simulink model "vestibular_3GDL"  (Simulink 7.7)
settings: Solver=ode45  StartTime=0.0  StopTime=30  RelTol=1e-3
values from neighbouring files (symbols this model uses):
  J = 0.02    [DCmotor.m]    (also in constantes_robot.m)
  Kb = 0.1    [DCmotor.m]    (also in constantes_robot.m)
  Kf = 0.2    [DCmotor.m]    (also in constantes_robot.m)
  Kff = 1/dcgain(dcm(1))    [DCmotor.m]    (also in constantes_robot.m)
  ki = str2double(get(hObject,'String'))    [interfaz_grafica.m]    (also in robot_simulacion.m = 8)
  ki1 = str2double(get(hObject,'String'))    [interfaz_grafica.m]    (also in robot_simulacion.m = 8)
  Km = 0.1    [DCmotor.m]    (also in constantes_robot.m)
  kp = str2double(get(hObject,'String'))    [interfaz_grafica.m]    (also in robot_simulacion.m = 2)
  L = 0.5    [DCmotor.m]    (also in constantes_robot.m)
  m = 1070    [constantesvestibular.m]    (also in modelo_vestibular.m)
  R = 2.0    (= 2)    [DCmotor.m]    (also in constantes_robot.m)
undefined symbols (not defined in the file or in its folder): articulacionX, articulacionY2, base, cabezalter, mastil, plataforma3, RootGround, RootPart, sigbuilder_block, vestibular_3GDL
libraries: mblibv1 x30, simulink_extras x3
settings Model: Creator=Ángel  LastModifiedBy=Ángel
settings SimMechanicsCC: VisOnUpdateDiagram=on  VisDuringSimulation=on

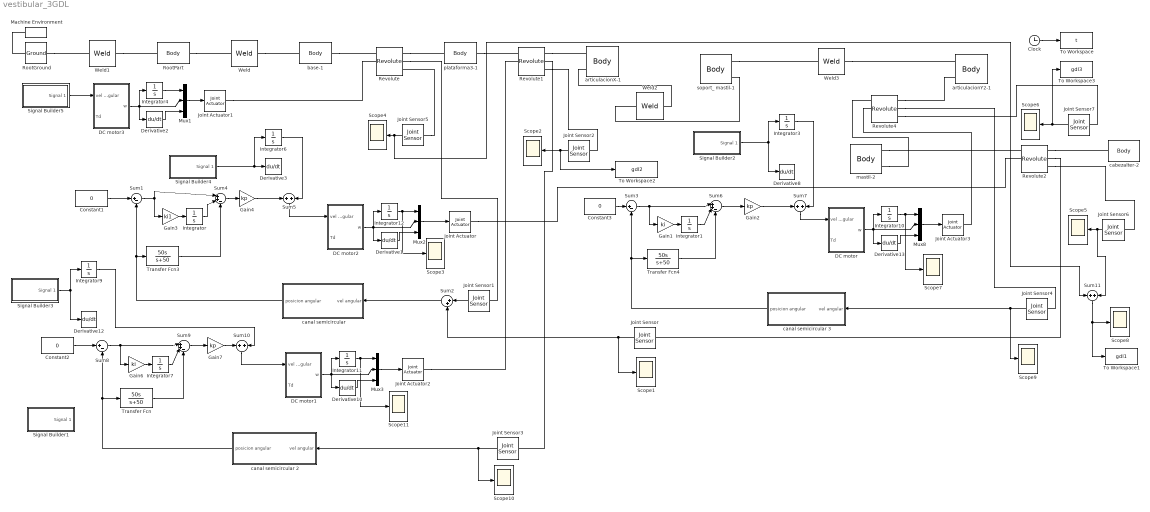
== system vestibular_3GDL ==
  Clock : Clock
      settings: Decimation=10
  Constant1 : Constant  Value=0
  Constant2 : Constant  Value=0
  Constant3 : Constant  Value=0
  DC motor : Subsystem
  DC motor1 : Subsystem
  DC motor2 : Subsystem
  DC motor3 : Subsystem
  Derivative{1..3,8,10,12..13} (7 alike) : Derivative
  Gain1 : Gain  Gain=ki
  Gain2 : Gain  Gain=kp
  Gain3 : Gain  Gain=ki1
  Gain4 : Gain  Gain=kp
  Gain6 : Gain  Gain=ki
  Gain7 : Gain  Gain=kp
  Integrator{,1,3..4,6..7,9..12} (10 alike) : Integrator
  Joint Actuator{,1..3} (4 alike) : mblibv1/Sensors &  Actuators/Joint Actuator  SystemSampleTime=-1  UpdateFromCAD=off  PhysicalDomain=Mechanical  PortType=blob  ActuationStyle=Motion  AngleUnits=rad  ArcVelocityUnits=rad/s  ArcAccelerationUnits=rad/s^2  CoordPositionUnits=m  VelocityUnits=m/s  AccelerationUnits=m/s^2  ForceUnits=N  TorqueUnits=N*m  ActiveIO=on  Width=3  DialogClass=MechanicalActuatorBlock  Primitive=R1  ReferenceFrame=Absolute (World)
  Joint Sensor : mblibv1/Sensors &  Actuators/Joint Sensor  SystemSampleTime=-1  UpdateFromCAD=off  PhysicalDomain=Mechanical  PortType=blob  Muxed=on  Pose=off  Angle=off  AngleUnits=rad  ArcVelocity=on  ArcVelocityUnits=rad/s  ArcAcceleration=off  ArcAccelerationUnits=deg/s^2  CoordPosition=on  CoordPositionUnits=m  Velocity=off  VelocityUnits=m/s  Acceleration=off  AccelerationUnits=m/s^2  Quaternion=on  QuaternionDT=off  QuaternionDDT=off  QuaternionUnits=off  OutputVector=[1]  ActiveIO=on  Width=1  DialogClass=MechanicalSensorBlock  Primitive=R1  Force=off  ForceUnits=N  Torque=off  TorqueUnits=N*m  ReferenceFrame=Absolute (World)  ReactionSensedSide=Base  ReactionReferenceFrame=Absolute (World)  ReactionForce=off  ReactionForceUnits=N  ReactionMoment=off  ReactionMomentUnits=N*m
  Joint Sensor1 : mblibv1/Sensors &  Actuators/Joint Sensor  SystemSampleTime=-1  UpdateFromCAD=off  PhysicalDomain=Mechanical  PortType=blob  Muxed=on  Pose=off  Angle=off  AngleUnits=rad  ArcVelocity=on  ArcVelocityUnits=rad/s  ArcAcceleration=off  ArcAccelerationUnits=rad/s^2  CoordPosition=on  CoordPositionUnits=m  Velocity=off  VelocityUnits=m/s  Acceleration=off  AccelerationUnits=m/s^2  Quaternion=on  QuaternionDT=off  QuaternionDDT=off  QuaternionUnits=off  OutputVector=[1]  ActiveIO=on  Width=1  DialogClass=MechanicalSensorBlock  Primitive=R1  Force=off  ForceUnits=N  Torque=off  TorqueUnits=N*m  ReferenceFrame=Absolute (World)  ReactionSensedSide=Base  ReactionReferenceFrame=Absolute (World)  ReactionForce=off  ReactionForceUnits=N  ReactionMoment=off  ReactionMomentUnits=N*m
  Joint Sensor{2,5..7} (4 alike) : mblibv1/Sensors &  Actuators/Joint Sensor  SystemSampleTime=-1  UpdateFromCAD=off  PhysicalDomain=Mechanical  PortType=blob  Muxed=on  Pose=off  Angle=on  AngleUnits=deg  ArcVelocity=off  ArcVelocityUnits=rad/s  ArcAcceleration=off  ArcAccelerationUnits=rad/s^2  CoordPosition=on  CoordPositionUnits=m  Velocity=off  VelocityUnits=m/s  Acceleration=off  AccelerationUnits=m/s^2  Quaternion=on  QuaternionDT=off  QuaternionDDT=off  QuaternionUnits=off  OutputVector=[1]  ActiveIO=on  Width=1  DialogClass=MechanicalSensorBlock  Primitive=R1  Force=off  ForceUnits=N  Torque=off  TorqueUnits=N*m  ReferenceFrame=Absolute (World)  ReactionSensedSide=Base  ReactionReferenceFrame=Absolute (World)  ReactionForce=off  ReactionForceUnits=N  ReactionMoment=off  ReactionMomentUnits=N*m
  Joint Sensor3 : mblibv1/Sensors &  Actuators/Joint Sensor  SystemSampleTime=-1  UpdateFromCAD=off  PhysicalDomain=Mechanical  PortType=blob  Muxed=on  Pose=off  Angle=off  AngleUnits=rad  ArcVelocity=on  ArcVelocityUnits=rad/s  ArcAcceleration=off  ArcAccelerationUnits=rad/s^2  CoordPosition=on  CoordPositionUnits=m  Velocity=off  VelocityUnits=m/s  Acceleration=off  AccelerationUnits=m/s^2  Quaternion=on  QuaternionDT=off  QuaternionDDT=off  QuaternionUnits=off  OutputVector=[1]  ActiveIO=on  Width=1  DialogClass=MechanicalSensorBlock  Primitive=R1  Force=off  ForceUnits=N  Torque=off  TorqueUnits=N*m  ReferenceFrame=Absolute (World)  ReactionSensedSide=Base  ReactionReferenceFrame=Absolute (World)  ReactionForce=off  ReactionForceUnits=N  ReactionMoment=off  ReactionMomentUnits=N*m
  Joint Sensor4 : mblibv1/Sensors &  Actuators/Joint Sensor  SystemSampleTime=-1  UpdateFromCAD=off  PhysicalDomain=Mechanical  PortType=blob  Muxed=on  Pose=off  Angle=off  AngleUnits=rad  ArcVelocity=on  ArcVelocityUnits=rad/s  ArcAcceleration=off  ArcAccelerationUnits=rad/s^2  CoordPosition=on  CoordPositionUnits=m  Velocity=off  VelocityUnits=m/s  Acceleration=off  AccelerationUnits=m/s^2  Quaternion=on  QuaternionDT=off  QuaternionDDT=off  QuaternionUnits=off  OutputVector=[1]  ActiveIO=on  Width=1  DialogClass=MechanicalSensorBlock  Primitive=R1  Force=off  ForceUnits=N  Torque=off  TorqueUnits=N*m  ReferenceFrame=Absolute (World)  ReactionSensedSide=Base  ReactionReferenceFrame=Absolute (World)  ReactionForce=off  ReactionForceUnits=N  ReactionMoment=off  ReactionMomentUnits=N*m
  Machine Environment : mblibv1/Bodies/Machine Environment  SystemSampleTime=-1  PortType=env  PhysicalDomain=Mechanical  DialogTemplateClass=MECH.MachineEnvironment  SyncWhenCopied=off  Gravity=[0 -9.81 0]  GravityUnits=m/s^2  GravityAsSignal=off  Dimensionality=Auto-detect  AnalysisType=Forward dynamics  LinearAssemblyTolerance=1e-3  LinearAssemblyToleranceUnits=m  AngularAssemblyTolerance=1e-3  AngularAssemblyToleranceUnits=rad  ConstraintSolverType=Stabilizing  ConstraintRelTolerance=1e-4  ConstraintAbsTolerance=1e-4  UseRobustSingularityHandling=off  RedundancyAnalysisToleranceType=Automatically select tolerance  RedundancyAnalysisTolerance=1e-14  StatePerturbationType=Fixed  PerturbationSize=1e-5  VisualizeMachine=on  BodyVisualizationType=Use model default body geometries  BodyColorSelMode=Use model default  DefaultBodyColor=[1 0 0]
  Mux{1..3,8} (4 alike) : Mux  Inputs=3
  Revolute : mblibv1/Joints/Revolute  PhysicalDomain=mechanical  SubClassName=Unknown  LeftPortType=blob  RightPortType=blob  LConnTagsString=__newl0|SA1|SA2  RConnTagsString=__newr0|SA1|SA2  UpdateFromCAD=on  PMImportedID=base-1:-:plataforma3-1  NumSAPorts=4  CutJoint=off  MarkAsCut=off  Primitives=prismatic  PrimitiveProps=R1$World$[-0.196775,0.962005,-0.189279]$revolute  DialogClass=JointBlock  R1Axis=[-0.196775,0.962005,-0.189279]
  Revolute1 : mblibv1/Joints/Revolute  PhysicalDomain=mechanical  SubClassName=Unknown  LeftPortType=blob  RightPortType=blob  LConnTagsString=__newl0|SA1|SA2  RConnTagsString=__newr0|SA1|SA2  UpdateFromCAD=on  PMImportedID=articulacionX-1:-:plataforma3-1  NumSAPorts=4  CutJoint=off  MarkAsCut=off  Primitives=prismatic  PrimitiveProps=R1$World$[-0.092947,-0.210487,-0.973168]$revolute  DialogClass=JointBlock  R1Axis=[-0.092947,-0.210487,-0.973168]
  Revolute2 : mblibv1/Joints/Revolute  PhysicalDomain=mechanical  SubClassName=Unknown  LeftPortType=blob  RightPortType=blob  LConnTagsString=__newl0|SA1|SA2  RConnTagsString=__newr0|SA1|SA2  UpdateFromCAD=on  PMImportedID=cabezalter-2:-:mastil-2  NumSAPorts=4  CutJoint=off  MarkAsCut=off  Primitives=prismatic  PrimitiveProps=R1$World$[-0.196775,0.962005,-0.189279]$revolute  DialogClass=JointBlock  R1Axis=[-0.196775,0.962005,-0.189279]
  Revolute4 : mblibv1/Joints/Revolute  PhysicalDomain=mechanical  SubClassName=Unknown  LeftPortType=blob  RightPortType=blob  LConnTagsString=__newl0|SA1|SA2  RConnTagsString=__newr0|SA1|SA2  UpdateFromCAD=on  PMImportedID=articulacionY2-1:-:mastil-2  NumSAPorts=4  CutJoint=off  MarkAsCut=off  Primitives=prismatic  PrimitiveProps=R1$World$[-0.976033,-0.173903,0.130834]$revolute  DialogClass=JointBlock  R1Axis=[-0.976033,-0.173903,0.130834]
  RootGround : mblibv1/Bodies/Ground  SystemSampleTime=-1  UpdateFromCAD=on  PMImportedID=RootGround  LeftPortType=env  RightPortType=workingframe  PhysicalDomain=Mechanical  DialogClass=GroundBlock  CoordPosition=[-0.906757,1.13031,1.7432]  CoordPositionUnits=m  StateVectorMgrId=-1  MachineId=[0 0]  ShowEnvPort=on
  RootPart : mblibv1/Bodies/Body  PhysicalDomain=mechanical  SubClassName=Unknown  LeftPortType=workingframe  RightPortType=workingframe  LConnTagsString=CS3  RConnTagsString=CS2  UpdateFromCAD=on  PMImportedID=vestibular_3GDL/RootPart  DialogClass=MechanicalBodyBlock  Mass=0  MassUnits=kg  InertiaUnits=kg*m^2  Inertia=[0,0,0;0,0,0;0,0,0]  Shape=Cylinder  ShapeDims=[1 1]  ShapeUnits=m  ShapeUse=false  Density=1  DensityUnits=kg/m^3  DensityUse=false  GraphicsMode=MACHINE_DEFAULT  BodyColorSelMode=MACHINE_DEFAULT  BodyColor=[1;0;0]  AttachedToCS=CS1  CG=Right$CG$[-0.906757 1.13031 1.7432]$WORLD$WORLD$m$[1 0 0;0 1 0;0 0 1]$3x3 Transform$rad$WORLD$false$vestibular_3GDL/RootPart::CG(AUTOGEN)  WorkingFrames=Right$CS1$[0 0 0]$WORLD$WORLD$m$[1 0 0;0 1 0;0 0 1]$3x3 Transform$rad$WORLD$false$vestibular_3GDL/RootPart::CS1(AUTOGEN)#Right$CS2$[-0.890894 1.04605 1.76218]$WORLD$WORLD$m$[1 0 0;0 1 0;0 0 1]$3x3 Transform$rad$WORLD$true$base-1:-:vestibular_3GDL/RootPart::vestibular_3GDL/RootPart(AUTOGEN)#Left$CS3$[-0.906757 1.13031 1.7432]$WORLD$WORLD$m$[1 0 0;0 1 0;0 0 1]$3x3 Transform$rad$WORLD$true$RootGround:-:vestibular_3GDL/RootPart::vestibular_3GDL/RootPart(AUTOGEN)  CGPos=[-0.906757 1.13031 1.7432]  CGRot=[1 0 0;0 1 0;0 0 1]  CS0Pos=[]  CS0Rot=[]  CS1Pos=[0 0 0]  CS1Rot=[1 0 0;0 1 0;0 0 1]  CS2Pos=[-0.890894 1.04605 1.76218]  CS2Rot=[1 0 0;0 1 0;0 0 1]  CS3Pos=[-0.906757 1.13031 1.7432]  CS3Rot=[1 0 0;0 1 0;0 0 1]  CS4Pos=[]  CS4Rot=[]  CS5Pos=[]  CS5Rot=[]  CS6Pos=[]  CS6Rot=[]  CS7Pos=[]  CS7Rot=[]  CS8Pos=[]  CS8Rot=[]  CS9Pos=[]  CS9Rot=[]  CS10Pos=[]  CS10Rot=[]  CS11Pos=[]  CS11Rot=[]  CS12Pos=[]  CS12Rot=[]  CS13Pos=[]  CS13Rot=[]  CS14Pos=[]  CS14Rot=[]  CS15Pos=[]  CS15Rot=[]  CS16Pos=[]  CS16Rot=[]  CS17Pos=[]  CS17Rot=[]  CS18Pos=[]  CS18Rot=[]  CS19Pos=[]  CS19Rot=[]  CS20Pos=[]  CS20Rot=[]
  Scope{1..11} (11 alike) : Scope
      Scope1 settings: TimeRange=2.754662840746054  YMin=-4e-006  YMax=6e-006
      Scope10 settings: TimeRange=2.754662840746054  YMin=-4e-006  YMax=6e-006  SaveName=ScopeData9
      Scope11 settings: TimeRange=2.754662840746054  YMin=-4e-006  YMax=6e-006  SaveName=ScopeData10
      Scope2 settings: TimeRange=2.754662840746054  YMin=-4e-006  YMax=6e-006  SaveName=ScopeData3
      Scope3 settings: TimeRange=2.754662840746054  YMin=-4e-006  YMax=6e-006  SaveName=ScopeData2
      Scope4 settings: TimeRange=2.754662840746054  YMin=-4e-006  YMax=6e-006  SaveName=ScopeData4
      Scope5 settings: TimeRange=2.754662840746054  YMin=-4e-006  YMax=6e-006  SaveName=ScopeData5
      Scope6 settings: TimeRange=2.754662840746054  YMin=-4e-006  YMax=6e-006  SaveName=ScopeData7
      Scope7 settings: TimeRange=2.754662840746054  YMin=-4e-006  YMax=6e-006  SaveName=ScopeData6
      Scope8 settings: TimeRange=2.754662840746054  YMin=-4e-006  YMax=6e-006  SaveName=ScopeData11
      Scope9 settings: TimeRange=2.754662840746054  YMin=-4e-006  YMax=6e-006  SaveName=ScopeData8
  Signal Builder1 : Subsystem  Tag=STV Subsys  LoadFcn=sigbuilder_block('load');  StartFcn=sigbuilder_block('start');  StopFcn=sigbuilder_block('stop');  ClipboardFcn=sigbuilder_block('clipboard');  mask(Sigbuilder block){}
      mask help: Create and generate interchangeable groups of signals whose waveforms are piecewise linear.
      mask init:
      | if ~strcmp(get_param(bdroot(gcbh),'SimulationStatus'),'stopped') tuvar = sigbuilder_block('maskInit'); end
      settings: CopyFcn=sigbuilder_block('copy');  DeleteFcn=sigbuilder_block('delete');  ModelCloseFcn=sigbuilder_block('modelClose');  PreSaveFcn=sigbuilder_block('preSave');  NameChangeFcn=sigbuilder_block('namechange');  OpenFcn=sigbuilder_block('open',[437.25 118.5 550.5 394.5 ]);  CloseFcn=sigbuilder_block('close');
      mask Display: plot(0, 0, 100, 100,[2, 2, 32, 32, 2], [68, 8, 8, 68, 68],[32, 2], [38, 38], [32, 19, 2],[53, 60, 44], [32, 17, 17, 2],[16, 16, 31, 31]);txt = getActiveGroup(gcbh);text(2, 100, txt,'verticalAlignment', 'top');
  Signal Builder2 : Subsystem  Tag=STV Subsys  LoadFcn=sigbuilder_block('load');  StartFcn=sigbuilder_block('start');  StopFcn=sigbuilder_block('stop');  ClipboardFcn=sigbuilder_block('clipboard');  mask(Sigbuilder block){}
      mask help: Create and generate interchangeable groups of signals whose waveforms are piecewise linear.
      mask init:
      | if ~strcmp(get_param(bdroot(gcbh),'SimulationStatus'),'stopped') tuvar = sigbuilder_block('maskInit'); end
      settings: CopyFcn=sigbuilder_block('copy');  DeleteFcn=sigbuilder_block('delete');  ModelCloseFcn=sigbuilder_block('modelClose');  PreSaveFcn=sigbuilder_block('preSave');  NameChangeFcn=sigbuilder_block('namechange');  OpenFcn=sigbuilder_block('open',[437.25 118.5 550.5 394.5 ]);  CloseFcn=sigbuilder_block('close');
      mask Display: plot(0, 0, 100, 100,[2, 2, 32, 32, 2], [68, 8, 8, 68, 68],[32, 2], [38, 38], [32, 19, 2],[53, 60, 44], [32, 17, 17, 2],[16, 16, 31, 31]);txt = getActiveGroup(gcbh);text(2, 100, txt,'verticalAlignment', 'top');
  Signal Builder3 : Subsystem  Tag=STV Subsys  LoadFcn=sigbuilder_block('load');  StartFcn=sigbuilder_block('start');  StopFcn=sigbuilder_block('stop');  ClipboardFcn=sigbuilder_block('clipboard');  mask(Sigbuilder block){}
      mask help: Create and generate interchangeable groups of signals whose waveforms are piecewise linear.
      mask init:
      | if ~strcmp(get_param(bdroot(gcbh),'SimulationStatus'),'stopped') tuvar = sigbuilder_block('maskInit'); end
      settings: CopyFcn=sigbuilder_block('copy');  DeleteFcn=sigbuilder_block('delete');  ModelCloseFcn=sigbuilder_block('modelClose');  PreSaveFcn=sigbuilder_block('preSave');  NameChangeFcn=sigbuilder_block('namechange');  OpenFcn=sigbuilder_block('open',[437.25 118.5 550.5 394.5 ]);  CloseFcn=sigbuilder_block('close');
      mask Display: plot(0, 0, 100, 100,[2, 2, 32, 32, 2], [68, 8, 8, 68, 68],[32, 2], [38, 38], [32, 19, 2],[53, 60, 44], [32, 17, 17, 2],[16, 16, 31, 31]);txt = getActiveGroup(gcbh);text(2, 100, txt,'verticalAlignment', 'top');
  Signal Builder4 : Subsystem  Tag=STV Subsys  LoadFcn=sigbuilder_block('load');  StartFcn=sigbuilder_block('start');  StopFcn=sigbuilder_block('stop');  ClipboardFcn=sigbuilder_block('clipboard');  mask(Sigbuilder block){}
      mask help: Create and generate interchangeable groups of signals whose waveforms are piecewise linear.
      mask init:
      | if ~strcmp(get_param(bdroot(gcbh),'SimulationStatus'),'stopped') tuvar = sigbuilder_block('maskInit'); end
      settings: CopyFcn=sigbuilder_block('copy');  DeleteFcn=sigbuilder_block('delete');  ModelCloseFcn=sigbuilder_block('modelClose');  PreSaveFcn=sigbuilder_block('preSave');  NameChangeFcn=sigbuilder_block('namechange');  OpenFcn=sigbuilder_block('open',[437.25 118.5 550.5 394.5 ]);  CloseFcn=sigbuilder_block('close');
      mask Display: plot(0, 0, 100, 100,[2, 2, 32, 32, 2], [68, 8, 8, 68, 68],[32, 2], [38, 38], [32, 19, 2],[53, 60, 44], [32, 17, 17, 2],[16, 16, 31, 31]);txt = getActiveGroup(gcbh);text(2, 100, txt,'verticalAlignment', 'top');
  Signal Builder5 : Subsystem  Tag=STV Subsys  LoadFcn=sigbuilder_block('load');  StartFcn=sigbuilder_block('start');  StopFcn=sigbuilder_block('stop');  ClipboardFcn=sigbuilder_block('clipboard');  mask(Sigbuilder block){}
      mask help: Create and generate interchangeable groups of signals whose waveforms are piecewise linear.
      mask init:
      | if ~strcmp(get_param(bdroot(gcbh),'SimulationStatus'),'stopped') tuvar = sigbuilder_block('maskInit'); end
      settings: CopyFcn=sigbuilder_block('copy');  DeleteFcn=sigbuilder_block('delete');  ModelCloseFcn=sigbuilder_block('modelClose');  PreSaveFcn=sigbuilder_block('preSave');  NameChangeFcn=sigbuilder_block('namechange');  OpenFcn=sigbuilder_block('open',[437.25 118.5 550.5 394.5 ]);  CloseFcn=sigbuilder_block('close');
      mask Display: plot(0, 0, 100, 100,[2, 2, 32, 32, 2], [68, 8, 8, 68, 68],[32, 2], [38, 38], [32, 19, 2],[53, 60, 44], [32, 17, 17, 2],[16, 16, 31, 31]);txt = getActiveGroup(gcbh);text(2, 100, txt,'verticalAlignment', 'top');
  Sum1 : Sum  Inputs=|+-
  Sum{5,7,10..11} (4 alike) : Sum  Inputs=+|+
  Sum2 : Sum  Inputs=|++
  Sum3 : Sum  Inputs=|+-
  Sum4 : Sum  Inputs=|++-
  Sum6 : Sum  Inputs=|++-
  Sum8 : Sum  Inputs=|+-
  Sum9 : Sum  Inputs=|++-
  To Workspace : ToWorkspace  VariableName=t  SampleTime=-1  SaveFormat=Array
  To Workspace1 : ToWorkspace  VariableName=gdl1  SampleTime=-1  SaveFormat=Array
  To Workspace2 : ToWorkspace  VariableName=gdl2  SampleTime=-1  SaveFormat=Array
  To Workspace3 : ToWorkspace  VariableName=gdl3  SampleTime=-1  SaveFormat=Array
  Transfer Fcn : TransferFcn  Numerator=[50 0]  Denominator=[1 50]
  Transfer Fcn3 : TransferFcn  Numerator=[50 0]  Denominator=[1 50]
  Transfer Fcn4 : TransferFcn  Numerator=[50 0]  Denominator=[1 50]
  Weld : mblibv1/Joints/Weld  PhysicalDomain=mechanical  SubClassName=Unknown  LeftPortType=blob  RightPortType=blob  LConnTagsString=__newl0  RConnTagsString=__newr0  UpdateFromCAD=on  PMImportedID=base-1:-:vestibular_3GDL/RootPart  NumSAPorts=0  CutJoint=off  MarkAsCut=off  Primitives=weld  PrimitiveProps=W$WORLD$[0.57735,0.57735,0.57735]$weld  DialogClass=JointBlock  WAxis=[0.57735,0.57735,0.57735]
  Weld1 : mblibv1/Joints/Weld  PhysicalDomain=mechanical  SubClassName=Unknown  LeftPortType=blob  RightPortType=blob  LConnTagsString=__newl0  RConnTagsString=__newr0  UpdateFromCAD=on  PMImportedID=RootGround:-:vestibular_3GDL/RootPart  NumSAPorts=0  CutJoint=off  MarkAsCut=off  Primitives=weld  PrimitiveProps=W$WORLD$[0.57735,0.57735,0.57735]$weld  DialogClass=JointBlock  WAxis=[0.57735,0.57735,0.57735]
  Weld2 : mblibv1/Joints/Weld  PhysicalDomain=mechanical  SubClassName=Unknown  LeftPortType=blob  RightPortType=blob  LConnTagsString=__newl0  RConnTagsString=__newr0  UpdateFromCAD=on  NumSAPorts=0  CutJoint=off  MarkAsCut=off  Primitives=weld  PrimitiveProps=W$WORLD$[0.57735,0.57735,0.57735]$weld  DialogClass=JointBlock  WAxis=[0.57735,0.57735,0.57735]
  Weld3 : mblibv1/Joints/Weld  PhysicalDomain=mechanical  SubClassName=Unknown  LeftPortType=blob  RightPortType=blob  LConnTagsString=__newl0  RConnTagsString=__newr0  UpdateFromCAD=on  NumSAPorts=0  CutJoint=off  MarkAsCut=off  Primitives=weld  PrimitiveProps=W$WORLD$[0.57735,0.57735,0.57735]$weld  DialogClass=JointBlock  WAxis=[0.57735,0.57735,0.57735]
  articulacionX-1 : mblibv1/Bodies/Body  PhysicalDomain=mechanical  SubClassName=Unknown  LeftPortType=workingframe  RightPortType=workingframe  LConnTagsString=CS2|CS3  UpdateFromCAD=on  PMImportedID=articulacionX-1  DialogClass=MechanicalBodyBlock  Mass=0.449248  MassUnits=kg  InertiaUnits=kg*m^2  Inertia=[0.00184415,0,0;0,0.00184415,0;0,0,0.000148165]  Shape=Cylinder  ShapeDims=[1 1]  ShapeUnits=m  ShapeUse=false  Density=1  DensityUnits=kg/m^3  DensityUse=false  GraphicsMode=GFXFILE  GraphicsFileName=vestibular_3GDL - articulacionX-1.STL  BodyColorSelMode=COLORPALETTE  BodyColor=[0;0.752941;0]  AttachedToCS=CS1  CG=Right$CG$[-0.929385 1.23548 1.71442]$WORLD$WORLD$m$[0.747256 0.658004 -0.092947;0.631181 -0.746529 -0.210487;-0.207889 0.0986216 -0.973168]$3x3 Transform$rad$WORLD$false$articulacionX-1::CG(AUTOGEN)  WorkingFrames=Right$CS1$[-0.919161 1.25863 1.82147]$WORLD$WORLD$m$[0.747256 0.658004 -0.092947;0.631181 -0.746529 -0.210487;-0.207889 0.0986216 -0.973168]$3x3 Transform$rad$WORLD$false$articulacionX-1::CS1(AUTOGEN)#Left$CS2$[-0.932639 1.22811 1.68036]$WORLD$WORLD$m$[1 0 0;0 1 0;0 0 1]$3x3 Transform$rad$WORLD$true$articulacionX-1:-:plataforma3-1::articulacionX-1(AUTOGEN)#Left$CS3$[-0.93961 1.21232 1.60737]$WORLD$WORLD$m$[1 0 0;0 1 0;0 0 1]$3x3 Transform$rad$WORLD$true$articulacionX-1:-:soport_ mastil-1::articulacionX-1(AUTOGEN)  CGPos=[-0.929385 1.23548 1.71442]  CGRot=[0.747256 0.658004 -0.092947;0.631181 -0.746529 -0.210487;-0.207889 0.0986216 -0.973168]  CS0Pos=[]  CS0Rot=[]  CS1Pos=[-0.919161 1.25863 1.82147]  CS1Rot=[0.747256 0.658004 -0.092947;0.631181 -0.746529 -0.210487;-0.207889 0.0986216 -0.973168]  CS2Pos=[-0.932639 1.22811 1.68036]  CS2Rot=[1 0 0;0 1 0;0 0 1]  CS3Pos=[-0.93961 1.21232 1.60737]  CS3Rot=[1 0 0;0 1 0;0 0 1]  CS4Pos=[]  CS4Rot=[]  CS5Pos=[]  CS5Rot=[]  CS6Pos=[]  CS6Rot=[]  CS7Pos=[]  CS7Rot=[]  CS8Pos=[]  CS8Rot=[]  CS9Pos=[]  CS9Rot=[]  CS10Pos=[]  CS10Rot=[]  CS11Pos=[]  CS11Rot=[]  CS12Pos=[]  CS12Rot=[]  CS13Pos=[]  CS13Rot=[]  CS14Pos=[]  CS14Rot=[]  CS15Pos=[]  CS15Rot=[]  CS16Pos=[]  CS16Rot=[]  CS17Pos=[]  CS17Rot=[]  CS18Pos=[]  CS18Rot=[]  CS19Pos=[]  CS19Rot=[]  CS20Pos=[]  CS20Rot=[]
  articulacionY2-1 : mblibv1/Bodies/Body  PhysicalDomain=mechanical  SubClassName=Unknown  LeftPortType=workingframe  RightPortType=workingframe  LConnTagsString=CS2|CS3  UpdateFromCAD=on  PMImportedID=articulacionY2-1  DialogClass=MechanicalBodyBlock  Mass=0.409978  MassUnits=kg  InertiaUnits=kg*m^2  Inertia=[0.00142936,0,0;0,0.00142936,0;0,0,0.000135894]  Shape=Cylinder  ShapeDims=[1 1]  ShapeUnits=m  ShapeUse=false  Density=1  DensityUnits=kg/m^3  DensityUse=false  GraphicsMode=GFXFILE  GraphicsFileName=vestibular_3GDL - articulacionY2-1.STL  BodyColorSelMode=COLORPALETTE  BodyColor=[0;0.752941;0]  AttachedToCS=CS1  CG=Right$CG$[-0.95595 1.36535 1.68887]$WORLD$WORLD$m$[-0.0960397 -0.195284 0.976033;-0.195284 0.965206 0.173903;-0.976033 -0.173903 -0.130834]$3x3 Transform$rad$WORLD$false$articulacionY2-1::CG(AUTOGEN)  WorkingFrames=Right$CS1$[-1.05355 1.34796 1.70195]$WORLD$WORLD$m$[-0.0960397 -0.195284 0.976033;-0.195284 0.965206 0.173903;-0.976033 -0.173903 -0.130834]$3x3 Transform$rad$WORLD$false$articulacionY2-1::CS1(AUTOGEN)#Left$CS2$[-0.858347 1.38274 1.67578]$WORLD$WORLD$m$[1 0 0;0 1 0;0 0 1]$3x3 Transform$rad$WORLD$true$articulacionY2-1:-:soport_ mastil-1::articulacionY2-1(AUTOGEN)#Left$CS3$[-1.00475 1.35665 1.69541]$WORLD$WORLD$m$[1 0 0;0 1 0;0 0 1]$3x3 Transform$rad$WORLD$true$articulacionY2-1:-:mastil-2::articulacionY2-1(AUTOGEN)  CGPos=[-0.95595 1.36535 1.68887]  CGRot=[-0.0960397 -0.195284 0.976033;-0.195284 0.965206 0.173903;-0.976033 -0.173903 -0.130834]  CS0Pos=[]  CS0Rot=[]  CS1Pos=[-1.05355 1.34796 1.70195]  CS1Rot=[-0.0960397 -0.195284 0.976033;-0.195284 0.965206 0.173903;-0.976033 -0.173903 -0.130834]  CS2Pos=[-0.858347 1.38274 1.67578]  CS2Rot=[1 0 0;0 1 0;0 0 1]  CS3Pos=[-1.00475 1.35665 1.69541]  CS3Rot=[1 0 0;0 1 0;0 0 1]  CS4Pos=[]  CS4Rot=[]  CS5Pos=[]  CS5Rot=[]  CS6Pos=[]  CS6Rot=[]  CS7Pos=[]  CS7Rot=[]  CS8Pos=[]  CS8Rot=[]  CS9Pos=[]  CS9Rot=[]  CS10Pos=[]  CS10Rot=[]  CS11Pos=[]  CS11Rot=[]  CS12Pos=[]  CS12Rot=[]  CS13Pos=[]  CS13Rot=[]  CS14Pos=[]  CS14Rot=[]  CS15Pos=[]  CS15Rot=[]  CS16Pos=[]  CS16Rot=[]  CS17Pos=[]  CS17Rot=[]  CS18Pos=[]  CS18Rot=[]  CS19Pos=[]  CS19Rot=[]  CS20Pos=[]  CS20Rot=[]
  base-1 : mblibv1/Bodies/Body  PhysicalDomain=mechanical  SubClassName=Unknown  LeftPortType=workingframe  RightPortType=workingframe  LConnTagsString=CS2  RConnTagsString=CS3  UpdateFromCAD=on  PMImportedID=base-1  DialogClass=MechanicalBodyBlock  Mass=19.3806  MassUnits=kg  InertiaUnits=kg*m^2  Inertia=[1.44455,-0.00802996,0.0117219;-0.00802996,1.54377,0.000942488;0.0117219,0.000942488,2.98379]  Shape=Cylinder  ShapeDims=[1 1]  ShapeUnits=m  ShapeUse=false  Density=1  DensityUnits=kg/m^3  DensityUse=false  GraphicsMode=GFXFILE  GraphicsFileName=vestibular_3GDL - base-1.STL  BodyColorSelMode=COLORPALETTE  BodyColor=[0.25098;0.25098;0.25098]  AttachedToCS=CS1  CG=Right$CG$[-0.890894 1.04605 1.76218]$WORLD$WORLD$m$[0.139887 -0.970418 -0.196775;-0.163531 -0.218643 0.962005;-0.97657 -0.102393 -0.189279]$3x3 Transform$rad$WORLD$false$base-1::CG(AUTOGEN)  WorkingFrames=Right$CS1$[-0.888063 1.03346 1.75417]$WORLD$WORLD$m$[0.139887 -0.970418 -0.196775;-0.163531 -0.218643 0.962005;-0.97657 -0.102393 -0.189279]$3x3 Transform$rad$WORLD$false$base-1::CS1(AUTOGEN)#Left$CS2$[-0.890894 1.04605 1.76218]$WORLD$WORLD$m$[1 0 0;0 1 0;0 0 1]$3x3 Transform$rad$WORLD$true$base-1:-:vestibular_3GDL/RootPart::base-1(AUTOGEN)#Right$CS3$[-0.891998 1.0527 1.75038]$WORLD$WORLD$m$[1 0 0;0 1 0;0 0 1]$3x3 Transform$rad$WORLD$true$base-1:-:plataforma3-1::base-1(AUTOGEN)  CGPos=[-0.890894 1.04605 1.76218]  CGRot=[0.139887 -0.970418 -0.196775;-0.163531 -0.218643 0.962005;-0.97657 -0.102393 -0.189279]  CS0Pos=[]  CS0Rot=[]  CS1Pos=[-0.888063 1.03346 1.75417]  CS1Rot=[0.139887 -0.970418 -0.196775;-0.163531 -0.218643 0.962005;-0.97657 -0.102393 -0.189279]  CS2Pos=[-0.890894 1.04605 1.76218]  CS2Rot=[1 0 0;0 1 0;0 0 1]  CS3Pos=[-0.891998 1.0527 1.75038]  CS3Rot=[1 0 0;0 1 0;0 0 1]  CS4Pos=[]  CS4Rot=[]  CS5Pos=[]  CS5Rot=[]  CS6Pos=[]  CS6Rot=[]  CS7Pos=[]  CS7Rot=[]  CS8Pos=[]  CS8Rot=[]  CS9Pos=[]  CS9Rot=[]  CS10Pos=[]  CS10Rot=[]  CS11Pos=[]  CS11Rot=[]  CS12Pos=[]  CS12Rot=[]  CS13Pos=[]  CS13Rot=[]  CS14Pos=[]  CS14Rot=[]  CS15Pos=[]  CS15Rot=[]  CS16Pos=[]  CS16Rot=[]  CS17Pos=[]  CS17Rot=[]  CS18Pos=[]  CS18Rot=[]  CS19Pos=[]  CS19Rot=[]  CS20Pos=[]  CS20Rot=[]
  cabezalter-2 : mblibv1/Bodies/Body  PhysicalDomain=mechanical  SubClassName=Unknown  LeftPortType=workingframe  RightPortType=workingframe  LConnTagsString=CS2  UpdateFromCAD=on  PMImportedID=cabezalter-2  DialogClass=MechanicalBodyBlock  Mass=2.12992  MassUnits=kg  InertiaUnits=kg*m^2  Inertia=[0.00545804,-3.68059e-009,-2.35881e-008;-3.68059e-009,0.00566829,-5.55414e-005;-2.35881e-008,-5.55414e-005,0.00533957]  Shape=Cylinder  ShapeDims=[1 1]  ShapeUnits=m  ShapeUse=false  Density=1  DensityUnits=kg/m^3  DensityUse=false  GraphicsMode=GFXFILE  GraphicsFileName=vestibular_3GDL - cabezalter-2.STL  BodyColorSelMode=COLORPALETTE  BodyColor=[0.988235;0.737255;0.517647]  AttachedToCS=CS1  CG=Right$CG$[-1.07939 1.96891 1.57114]$WORLD$WORLD$m$[0.980265 -0.196775 -0.0189833;0.196775 0.962005 0.189279;-0.0189833 -0.189279 0.98174]$3x3 Transform$rad$WORLD$false$cabezalter-2::CG(AUTOGEN)  WorkingFrames=Right$CS1$[-1.07902 1.96701 1.57049]$WORLD$WORLD$m$[0.980265 -0.196775 -0.0189833;0.196775 0.962005 0.189279;-0.0189833 -0.189279 0.98174]$3x3 Transform$rad$WORLD$false$cabezalter-2::CS1(AUTOGEN)#Left$CS2$[-1.06811 1.91369 1.58098]$WORLD$WORLD$m$[1 0 0;0 1 0;0 0 1]$3x3 Transform$rad$WORLD$true$cabezalter-2:-:mastil-2::cabezalter-2(AUTOGEN)  CGPos=[-1.07939 1.96891 1.57114]  CGRot=[0.980265 -0.196775 -0.0189833;0.196775 0.962005 0.189279;-0.0189833 -0.189279 0.98174]  CS0Pos=[]  CS0Rot=[]  CS1Pos=[-1.07902 1.96701 1.57049]  CS1Rot=[0.980265 -0.196775 -0.0189833;0.196775 0.962005 0.189279;-0.0189833 -0.189279 0.98174]  CS2Pos=[-1.06811 1.91369 1.58098]  CS2Rot=[1 0 0;0 1 0;0 0 1]  CS3Pos=[]  CS3Rot=[]  CS4Pos=[]  CS4Rot=[]  CS5Pos=[]  CS5Rot=[]  CS6Pos=[]  CS6Rot=[]  CS7Pos=[]  CS7Rot=[]  CS8Pos=[]  CS8Rot=[]  CS9Pos=[]  CS9Rot=[]  CS10Pos=[]  CS10Rot=[]  CS11Pos=[]  CS11Rot=[]  CS12Pos=[]  CS12Rot=[]  CS13Pos=[]  CS13Rot=[]  CS14Pos=[]  CS14Rot=[]  CS15Pos=[]  CS15Rot=[]  CS16Pos=[]  CS16Rot=[]  CS17Pos=[]  CS17Rot=[]  CS18Pos=[]  CS18Rot=[]  CS19Pos=[]  CS19Rot=[]  CS20Pos=[]  CS20Rot=[]
  canal semicircular : Subsystem
  canal semicircular 2 : Subsystem
  canal semicircular 3 : Subsystem
  mastil-2 : mblibv1/Bodies/Body  PhysicalDomain=mechanical  SubClassName=Unknown  LeftPortType=workingframe  RightPortType=workingframe  RConnTagsString=CS2|CS3  UpdateFromCAD=on  PMImportedID=mastil-2  DialogClass=MechanicalBodyBlock  Mass=3.50962  MassUnits=kg  InertiaUnits=kg*m^2  Inertia=[0.075228,0,0;0,0.0750951,0;0,0,0.00440334]  Shape=Cylinder  ShapeDims=[1 1]  ShapeUnits=m  ShapeUse=false  Density=1  DensityUnits=kg/m^3  DensityUse=false  GraphicsMode=GFXFILE  GraphicsFileName=vestibular_3GDL - mastil-2.STL  BodyColorSelMode=COLORPALETTE  BodyColor=[0;0;1]  AttachedToCS=CS1  CG=Right$CG$[-0.996339 1.5628 1.65002]$WORLD$WORLD$m$[0.976033 0.092947 0.196775;0.173903 0.210487 -0.962005;-0.130834 0.973168 0.189279]$3x3 Transform$rad$WORLD$false$mastil-2::CG(AUTOGEN)  WorkingFrames=Right$CS1$[-1.02876 1.72129 1.61883]$WORLD$WORLD$m$[0.976033 0.092947 0.196775;0.173903 0.210487 -0.962005;-0.130834 0.973168 0.189279]$3x3 Transform$rad$WORLD$false$mastil-2::CS1(AUTOGEN)#Right$CS2$[-1.06811 1.91369 1.58098]$WORLD$WORLD$m$[1 0 0;0 1 0;0 0 1]$3x3 Transform$rad$WORLD$true$cabezalter-2:-:mastil-2::mastil-2(AUTOGEN)#Right$CS3$[-1.00475 1.35665 1.69541]$WORLD$WORLD$m$[1 0 0;0 1 0;0 0 1]$3x3 Transform$rad$WORLD$true$articulacionY2-1:-:mastil-2::mastil-2(AUTOGEN)  CGPos=[-0.996339 1.5628 1.65002]  CGRot=[0.976033 0.092947 0.196775;0.173903 0.210487 -0.962005;-0.130834 0.973168 0.189279]  CS0Pos=[]  CS0Rot=[]  CS1Pos=[-1.02876 1.72129 1.61883]  CS1Rot=[0.976033 0.092947 0.196775;0.173903 0.210487 -0.962005;-0.130834 0.973168 0.189279]  CS2Pos=[-1.06811 1.91369 1.58098]  CS2Rot=[1 0 0;0 1 0;0 0 1]  CS3Pos=[-1.00475 1.35665 1.69541]  CS3Rot=[1 0 0;0 1 0;0 0 1]  CS4Pos=[]  CS4Rot=[]  CS5Pos=[]  CS5Rot=[]  CS6Pos=[]  CS6Rot=[]  CS7Pos=[]  CS7Rot=[]  CS8Pos=[]  CS8Rot=[]  CS9Pos=[]  CS9Rot=[]  CS10Pos=[]  CS10Rot=[]  CS11Pos=[]  CS11Rot=[]  CS12Pos=[]  CS12Rot=[]  CS13Pos=[]  CS13Rot=[]  CS14Pos=[]  CS14Rot=[]  CS15Pos=[]  CS15Rot=[]  CS16Pos=[]  CS16Rot=[]  CS17Pos=[]  CS17Rot=[]  CS18Pos=[]  CS18Rot=[]  CS19Pos=[]  CS19Rot=[]  CS20Pos=[]  CS20Rot=[]
  plataforma3-1 : mblibv1/Bodies/Body  PhysicalDomain=mechanical  SubClassName=Unknown  LeftPortType=workingframe  RightPortType=workingframe  LConnTagsString=CS2  RConnTagsString=CS3  UpdateFromCAD=on  PMImportedID=plataforma3-1  DialogClass=MechanicalBodyBlock  Mass=40.7194  MassUnits=kg  InertiaUnits=kg*m^2  Inertia=[2.62975,0.0149464,-0.00326412;0.0149464,2.48143,0.0327264;-0.00326412,0.0327264,5.06129]  Shape=Cylinder  ShapeDims=[1 1]  ShapeUnits=m  ShapeUse=false  Density=1  DensityUnits=kg/m^3  DensityUse=false  GraphicsMode=GFXFILE  GraphicsFileName=vestibular_3GDL - plataforma3-1.STL  BodyColorSelMode=COLORPALETTE  BodyColor=[0.501961;0.501961;1]  AttachedToCS=CS1  CG=Right$CG$[-0.896029 1.08206 1.75298]$WORLD$WORLD$m$[0.976033 -0.092947 -0.196775;0.173903 -0.210487 0.962005;-0.130834 -0.973168 -0.189279]$3x3 Transform$rad$WORLD$false$plataforma3-1::CG(AUTOGEN)  WorkingFrames=Right$CS1$[-0.891998 1.0527 1.75038]$WORLD$WORLD$m$[0.976033 -0.092947 -0.196775;0.173903 -0.210487 0.962005;-0.130834 -0.973168 -0.189279]$3x3 Transform$rad$WORLD$false$plataforma3-1::CS1(AUTOGEN)#Left$CS2$[-0.891998 1.0527 1.75038]$WORLD$WORLD$m$[1 0 0;0 1 0;0 0 1]$3x3 Transform$rad$WORLD$true$base-1:-:plataforma3-1::plataforma3-1(AUTOGEN)#Right$CS3$[-0.932639 1.22811 1.68036]$WORLD$WORLD$m$[1 0 0;0 1 0;0 0 1]$3x3 Transform$rad$WORLD$true$articulacionX-1:-:plataforma3-1::plataforma3-1(AUTOGEN)  CGPos=[-0.896029 1.08206 1.75298]  CGRot=[0.976033 -0.092947 -0.196775;0.173903 -0.210487 0.962005;-0.130834 -0.973168 -0.189279]  CS0Pos=[]  CS0Rot=[]  CS1Pos=[-0.891998 1.0527 1.75038]  CS1Rot=[0.976033 -0.092947 -0.196775;0.173903 -0.210487 0.962005;-0.130834 -0.973168 -0.189279]  CS2Pos=[-0.891998 1.0527 1.75038]  CS2Rot=[1 0 0;0 1 0;0 0 1]  CS3Pos=[-0.932639 1.22811 1.68036]  CS3Rot=[1 0 0;0 1 0;0 0 1]  CS4Pos=[]  CS4Rot=[]  CS5Pos=[]  CS5Rot=[]  CS6Pos=[]  CS6Rot=[]  CS7Pos=[]  CS7Rot=[]  CS8Pos=[]  CS8Rot=[]  CS9Pos=[]  CS9Rot=[]  CS10Pos=[]  CS10Rot=[]  CS11Pos=[]  CS11Rot=[]  CS12Pos=[]  CS12Rot=[]  CS13Pos=[]  CS13Rot=[]  CS14Pos=[]  CS14Rot=[]  CS15Pos=[]  CS15Rot=[]  CS16Pos=[]  CS16Rot=[]  CS17Pos=[]  CS17Rot=[]  CS18Pos=[]  CS18Rot=[]  CS19Pos=[]  CS19Rot=[]  CS20Pos=[]  CS20Rot=[]
  soport_ mastil-1 : mblibv1/Bodies/Body  PhysicalDomain=mechanical  SubClassName=Unknown  LeftPortType=workingframe  RightPortType=workingframe  RConnTagsString=CS2|CS3  UpdateFromCAD=on  PMImportedID=soport_ mastil-1  DialogClass=MechanicalBodyBlock  Mass=1.00146  MassUnits=kg  InertiaUnits=kg*m^2  Inertia=[0.0110546,0,0;0,0.0131157,0;0,0,0.00857204]  Shape=Cylinder  ShapeDims=[1 1]  ShapeUnits=m  ShapeUse=false  Density=1  DensityUnits=kg/m^3  DensityUse=false  GraphicsMode=GFXFILE  GraphicsFileName=vestibular_3GDL - soport_ mastil-1.STL  BodyColorSelMode=COLORPALETTE  BodyColor=[1;1;0]  AttachedToCS=CS1  CG=Right$CG$[-0.938561 1.28034 1.70559]$WORLD$WORLD$m$[-0.092947 -0.196775 0.976033;-0.210487 0.962005 0.173903;-0.973168 -0.189279 -0.130834]$3x3 Transform$rad$WORLD$false$soport_ mastil-1::CG(AUTOGEN)  WorkingFrames=Right$CS1$[-1.01081 1.20547 1.83145]$WORLD$WORLD$m$[-0.092947 -0.196775 0.976033;-0.210487 0.962005 0.173903;-0.973168 -0.189279 -0.130834]$3x3 Transform$rad$WORLD$false$soport_ mastil-1::CS1(AUTOGEN)#Right$CS2$[-0.858347 1.38274 1.67578]$WORLD$WORLD$m$[1 0 0;0 1 0;0 0 1]$3x3 Transform$rad$WORLD$true$articulacionY2-1:-:soport_ mastil-1::soport_ mastil-1(AUTOGEN)#Right$CS3$[-0.93961 1.21232 1.60737]$WORLD$WORLD$m$[1 0 0;0 1 0;0 0 1]$3x3 Transform$rad$WORLD$true$articulacionX-1:-:soport_ mastil-1::soport_ mastil-1(AUTOGEN)  CGPos=[-0.938561 1.28034 1.70559]  CGRot=[-0.092947 -0.196775 0.976033;-0.210487 0.962005 0.173903;-0.973168 -0.189279 -0.130834]  CS0Pos=[]  CS0Rot=[]  CS1Pos=[-1.01081 1.20547 1.83145]  CS1Rot=[-0.092947 -0.196775 0.976033;-0.210487 0.962005 0.173903;-0.973168 -0.189279 -0.130834]  CS2Pos=[-0.858347 1.38274 1.67578]  CS2Rot=[1 0 0;0 1 0;0 0 1]  CS3Pos=[-0.93961 1.21232 1.60737]  CS3Rot=[1 0 0;0 1 0;0 0 1]  CS4Pos=[]  CS4Rot=[]  CS5Pos=[]  CS5Rot=[]  CS6Pos=[]  CS6Rot=[]  CS7Pos=[]  CS7Rot=[]  CS8Pos=[]  CS8Rot=[]  CS9Pos=[]  CS9Rot=[]  CS10Pos=[]  CS10Rot=[]  CS11Pos=[]  CS11Rot=[]  CS12Pos=[]  CS12Rot=[]  CS13Pos=[]  CS13Rot=[]  CS14Pos=[]  CS14Rot=[]  CS15Pos=[]  CS15Rot=[]  CS16Pos=[]  CS16Rot=[]  CS17Pos=[]  CS17Rot=[]  CS18Pos=[]  CS18Rot=[]  CS19Pos=[]  CS19Rot=[]  CS20Pos=[]  CS20Rot=[]
  wires:
  Joint Sensor/1 -> Scope1/1, Sum2/2
  canal semicircular/1(posicion angular) -> Sum1/2, Transfer Fcn3/1
  Sum2/1 -> canal semicircular/1(vel angular)
  Sum1/1 -> Gain3/1, Sum4/1
  Joint Sensor1/1 -> Sum2/1
  Gain3/1 -> Integrator/1
  Gain4/1 -> Sum5/1
  Constant1/1 -> Sum1/1
  Signal Builder4/1(Signal 1) -> Integrator6/1, Derivative3/1
  canal semicircular 3/1(posicion angular) -> Sum3/2, Transfer Fcn4/1
  Sum3/1 -> Gain1/1, Sum6/1
  Gain1/1 -> Integrator1/1
  Integrator1/1 -> Sum6/2
  Gain2/1 -> Sum7/1
  Joint Sensor4/1 -> Scope9/1, canal semicircular 3/1(vel angular)
  Constant3/1 -> Sum3/1
  Sum6/1 -> Gain2/1
  Signal Builder2/1(Signal 1) -> Integrator3/1, Derivative8/1
  canal semicircular 2/1(posicion angular) -> Sum8/2, Transfer Fcn/1
  Sum8/1 -> Sum9/1, Gain6/1
  Gain6/1 -> Integrator7/1
  Integrator7/1 -> Sum9/2
  Sum9/1 -> Gain7/1
  Gain7/1 -> Sum10/1
  Constant2/1 -> Sum8/1
  Joint Sensor3/1 -> Scope10/1, canal semicircular 2/1(vel angular)
  Signal Builder3/1(Signal 1) -> Integrator9/1, Derivative12/1
  DC motor/1(w) -> Derivative13/1, Mux8/2, Integrator10/1
  Derivative13/1 -> Mux8/3
  Integrator10/1 -> Mux8/1, Scope7/1
  DC motor1/1(w) -> Integrator11/1, Mux3/2, Derivative10/1
  Derivative10/1 -> Mux3/3
  Integrator11/1 -> Mux3/1, Scope11/1
  Sum10/1 -> DC motor1/1(vel angular)
  Mux3/1 -> Joint Actuator2/1
  DC motor2/1(w) -> Integrator12/1, Mux2/2, Derivative1/1
  Derivative1/1 -> Mux2/3
  Integrator12/1 -> Mux2/1, Scope3/1
  Sum5/1 -> DC motor2/1(vel angular)
  Mux2/1 -> Joint Actuator/1
  Sum7/1 -> DC motor/1(vel angular)
  Mux8/1 -> Joint Actuator3/1
  Integrator6/1 -> Sum5/2
  Integrator9/1 -> Sum10/2
  Transfer Fcn/1 -> Sum9/3
  Sum4/1 -> Gain4/1
  Transfer Fcn3/1 -> Sum4/3
  Integrator/1 -> Sum4/2
  Integrator3/1 -> Sum7/2
  Transfer Fcn4/1 -> Sum6/3
  Joint Sensor2/1 -> Scope2/1, To Workspace2/1
  Joint Sensor5/1 -> Scope4/1, Sum11/1
  Joint Sensor6/1 -> Scope5/1, Sum11/2
  Joint Sensor7/1 -> Scope6/1, To Workspace3/1
  Sum11/1 -> Scope8/1, To Workspace1/1
  DC motor3/1(w) -> Derivative2/1, Mux1/2, Integrator4/1
  Derivative2/1 -> Mux1/3
  Integrator4/1 -> Mux1/1
  Mux1/1 -> Joint Actuator1/1
  Signal Builder5/1(Signal 1) -> DC motor3/1(vel angular)
  Clock/1 -> To Workspace/1
  connections:
  RootPart/RConn1 -- Weld/LConn1
  Weld/RConn1 -- base-1/LConn1
  base-1/RConn1 -- Revolute/LConn1
  Revolute/RConn1 -- plataforma3-1/LConn1
  plataforma3-1/RConn1 -- Revolute1/LConn1
  Revolute1/RConn1 -- articulacionX-1/LConn1
  mastil-2/RConn1 -- Revolute2/LConn1
  Revolute2/RConn1 -- cabezalter-2/LConn1
  soport_ mastil-1/RConn1 -- Weld3/LConn1
  Weld3/RConn1 -- articulacionY2-1/LConn1
  mastil-2/RConn2 -- Revolute4/LConn1
  Revolute4/RConn1 -- articulacionY2-1/LConn2
  soport_ mastil-1/RConn2 -- Weld2/LConn1
  Weld2/RConn1 -- articulacionX-1/LConn2
  RootGround/RConn1 -- Weld1/LConn1
  Weld1/RConn1 -- RootPart/LConn1
  RootGround/LConn1 -- Machine Environment/RConn1
  Joint Actuator/RConn1 -- Revolute2/LConn2
  Revolute2/RConn2 -- Joint Sensor/LConn1
  Joint Actuator3/RConn1 -- Revolute4/LConn2
  Revolute4/RConn2 -- Joint Sensor4/LConn1
  Joint Actuator1/RConn1 -- Revolute/LConn2
  Revolute/RConn2 -- Joint Sensor1/LConn1
  Joint Actuator2/RConn1 -- Revolute1/LConn2
  Revolute1/RConn2 -- Joint Sensor3/LConn1
  Revolute1/RConn3 -- Joint Sensor2/LConn1
  Joint Sensor5/LConn1 -- Revolute/RConn3
  Revolute2/RConn3 -- Joint Sensor6/LConn1
  Revolute4/RConn3 -- Joint Sensor7/LConn1

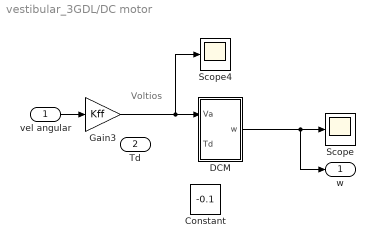
== system vestibular_3GDL/DC motor ==
  note: Voltios
  vel angular : Inport
  Td : Inport  Port=2
  Constant : Constant  Value=-0.1
  DCM : Subsystem
  Gain3 : Gain  Gain=Kff
  Scope : Scope
  Scope4 : Scope
  w : Outport
  wires:
  Gain3/1 -> DCM/1(Va), Scope4/1
  DCM/1(w) -> Scope/1, w/1
  vel angular/1 -> Gain3/1

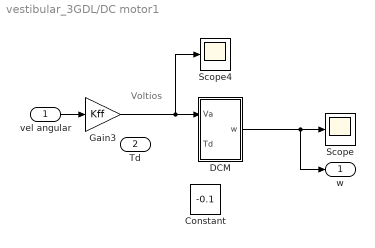
== system vestibular_3GDL/DC motor1 ==
  note: Voltios
  vel angular : Inport
  Td : Inport  Port=2
  Constant : Constant  Value=-0.1
  DCM : Subsystem
  Gain3 : Gain  Gain=Kff
  Scope : Scope
  Scope4 : Scope
  w : Outport
  wires:
  vel angular/1 -> Gain3/1
  DCM/1(w) -> w/1, Scope/1
  Gain3/1 -> Scope4/1, DCM/1(Va)

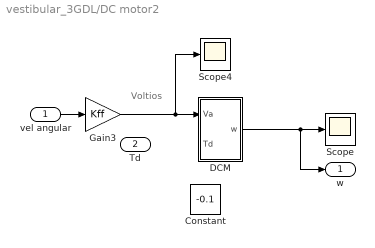
== system vestibular_3GDL/DC motor2 ==
  note: Voltios
  vel angular : Inport
  Td : Inport  Port=2
  Constant : Constant  Value=-0.1
  DCM : Subsystem
  Gain3 : Gain  Gain=Kff
  Scope : Scope
  Scope4 : Scope
  w : Outport
  wires:
  vel angular/1 -> Gain3/1
  DCM/1(w) -> w/1, Scope/1
  Gain3/1 -> Scope4/1, DCM/1(Va)

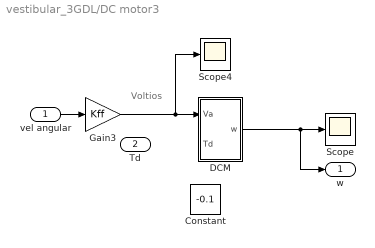
== system vestibular_3GDL/DC motor3 ==
  note: Voltios
  vel angular : Inport
  Td : Inport  Port=2
  Constant : Constant  Value=-0.1
  DCM : Subsystem
  Gain3 : Gain  Gain=Kff
  Scope : Scope
  Scope4 : Scope
  w : Outport
  wires:
  Gain3/1 -> DCM/1(Va), Scope4/1
  DCM/1(w) -> Scope/1, w/1
  vel angular/1 -> Gain3/1

== system vestibular_3GDL/Signal Builder1 ==
  Demux : Demux  Tag=STV Demux  Outputs=1
  FromWs : FromWorkspace  Tag=STV FromWs  VariableName=tuvar  SampleTime=0  SigBuilderData=DataTag1  VnvData=DataTag2
      SigBuilderData=|
      | common.afterFinalStr = 'Extrapolate'
      | common.sampleTime = 0
      | dataSet.timeRange = [0 20]
      | dataSet.name = 'Group 1'
      | sbobj.Groups.Name = 'Group 1'
      | sbobj.Groups.Signals.Name = 'Signal 1'
      | sbobj.Groups.Signals.XData = [0 0.98 1 2.04 4 5 6 7 8 9 20]
      | sbobj.Groups.Signals.YData = [0 0 0 1.74532925199 1.7417883396 -1.7418 1.7418 1.7418 -1.7418 0 0]
      | sbobj.Groups.TimeRange = [0 20]
  Signal 1 : Outport  Tag=STV Outport
  wires:
  Demux/1 -> Signal 1/1
  FromWs/1 -> Demux/1

== system vestibular_3GDL/Signal Builder2 ==
  Demux : Demux  Tag=STV Demux  Outputs=1
  FromWs : FromWorkspace  Tag=STV FromWs  VariableName=tuvar  SampleTime=0  SigBuilderData=DataTag3  VnvData=DataTag4
      SigBuilderData=|
      | common.afterFinalStr = 'Extrapolate'
      | common.sampleTime = 0
      | dataSet.timeRange = [0 20]
      | dataSet.name = 'Group 1'
      | sbobj.Groups.Name = 'Group 1'
      | sbobj.Groups.Signals.Name = 'Signal 1'
      | sbobj.Groups.Signals.XData = [0 1 4 5 6 12 13 20]
      | sbobj.Groups.Signals.YData = [0 1.5 1.5 0 -1.5 -1.5 0 0]
      | sbobj.Groups.TimeRange = [0 20]
  Signal 1 : Outport  Tag=STV Outport
  wires:
  Demux/1 -> Signal 1/1
  FromWs/1 -> Demux/1

== system vestibular_3GDL/Signal Builder3 ==
  Demux : Demux  Tag=STV Demux  Outputs=1
  FromWs : FromWorkspace  Tag=STV FromWs  VariableName=tuvar  SampleTime=0  SigBuilderData=DataTag5  VnvData=DataTag6
      SigBuilderData=|
      | common.afterFinalStr = 'Extrapolate'
      | common.sampleTime = 0
      | dataSet.timeRange = [0 20]
      | dataSet.name = 'Group 1'
      | sbobj.Groups.Name = 'Group 1'
      | sbobj.Groups.Signals.Name = 'Signal 1'
      | sbobj.Groups.Signals.XData = [0 1 4 5 6 12 13 20]
      | sbobj.Groups.Signals.YData = [0 1.5 1.5 0 -1.5 -1.5 0 0]
      | sbobj.Groups.TimeRange = [0 20]
  Signal 1 : Outport  Tag=STV Outport
  wires:
  Demux/1 -> Signal 1/1
  FromWs/1 -> Demux/1

== system vestibular_3GDL/Signal Builder4 ==
  Demux : Demux  Tag=STV Demux  Outputs=1
  FromWs : FromWorkspace  Tag=STV FromWs  VariableName=tuvar  SampleTime=0  SigBuilderData=DataTag7  VnvData=DataTag8
      SigBuilderData=|
      | common.afterFinalStr = 'Extrapolate'
      | common.sampleTime = 0
      | dataSet.timeRange = [0 20]
      | dataSet.name = 'Group 1'
      | sbobj.Groups.Name = 'Group 1'
      | sbobj.Groups.Signals.Name = 'Signal 1'
      | sbobj.Groups.Signals.XData = [0 1 4 5 6 12 13 20]
      | sbobj.Groups.Signals.YData = [0 1.5 1.5 0 -1.5 -1.5 0 0]
      | sbobj.Groups.TimeRange = [0 20]
  Signal 1 : Outport  Tag=STV Outport
  wires:
  FromWs/1 -> Demux/1
  Demux/1 -> Signal 1/1

== system vestibular_3GDL/Signal Builder5 ==
  Demux : Demux  Tag=STV Demux  Outputs=1
  FromWs : FromWorkspace  Tag=STV FromWs  VariableName=tuvar  SampleTime=0  SigBuilderData=DataTag9  VnvData=DataTag10
      SigBuilderData=|
      | common.afterFinalStr = 'Extrapolate'
      | common.sampleTime = 0
      | dataSet.timeRange = [0 10]
      | dataSet.name = 'Group 1'
      | sbobj.Groups.Name = 'Group 1'
      | sbobj.Groups.Signals.Name = 'Signal 1'
      | sbobj.Groups.Signals.XData = [0 1 2 3 4 5 8 10]
      | sbobj.Groups.Signals.YData = [0 1 1 0 0 0 0 0]
  Signal 1 : Outport  Tag=STV Outport
  wires:
  FromWs/1 -> Demux/1
  Demux/1 -> Signal 1/1

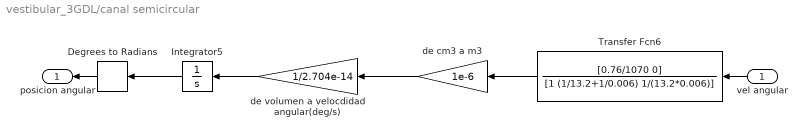
== system vestibular_3GDL/canal semicircular ==
  vel angular : Inport
  Degrees to Radians : simulink_extras/Transformations/Degrees to Radians  SystemSampleTime=-1
  Integrator5 : Integrator
  Transfer Fcn6 : TransferFcn  Numerator=[0.76/1070 0]  Denominator=[1 (1/13.2+1/0.006) 1/(13.2*0.006)]
  de cm3 a m3 : Gain  Gain=1e-6
  de volumen a velocdidad angular(deg/s) : Gain  Gain=1/2.704e-14
  posicion angular : Outport
  wires:
  Integrator5/1 -> Degrees to Radians/1
  de volumen a velocdidad angular(deg/s)/1 -> Integrator5/1
  de cm3 a m3/1 -> de volumen a velocdidad angular(deg/s)/1
  Transfer Fcn6/1 -> de cm3 a m3/1
  Degrees to Radians/1 -> posicion angular/1
  vel angular/1 -> Transfer Fcn6/1

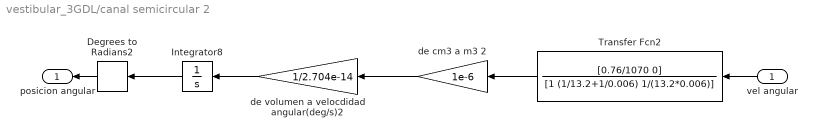
== system vestibular_3GDL/canal semicircular 2 ==
  vel angular : Inport
  Degrees to Radians2 : simulink_extras/Transformations/Degrees to Radians  SystemSampleTime=-1
  Integrator8 : Integrator
  Transfer Fcn2 : TransferFcn  Numerator=[0.76/1070 0]  Denominator=[1 (1/13.2+1/0.006) 1/(13.2*0.006)]
  de cm3 a m3 2 : Gain  Gain=1e-6
  de volumen a velocdidad angular(deg/s)2 : Gain  Gain=1/2.704e-14
  posicion angular : Outport
  wires:
  Transfer Fcn2/1 -> de cm3 a m3 2/1
  de cm3 a m3 2/1 -> de volumen a velocdidad angular(deg/s)2/1
  de volumen a velocdidad angular(deg/s)2/1 -> Integrator8/1
  Integrator8/1 -> Degrees to Radians2/1
  vel angular/1 -> Transfer Fcn2/1
  Degrees to Radians2/1 -> posicion angular/1

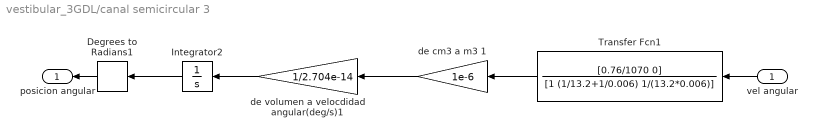
== system vestibular_3GDL/canal semicircular 3 ==
  vel angular : Inport
  Degrees to Radians1 : simulink_extras/Transformations/Degrees to Radians  SystemSampleTime=-1
  Integrator2 : Integrator
  Transfer Fcn1 : TransferFcn  Numerator=[0.76/1070 0]  Denominator=[1 (1/13.2+1/0.006) 1/(13.2*0.006)]
  de cm3 a m3 1 : Gain  Gain=1e-6
  de volumen a velocdidad angular(deg/s)1 : Gain  Gain=1/2.704e-14
  posicion angular : Outport
  wires:
  Transfer Fcn1/1 -> de cm3 a m3 1/1
  de cm3 a m3 1/1 -> de volumen a velocdidad angular(deg/s)1/1
  de volumen a velocdidad angular(deg/s)1/1 -> Integrator2/1
  Integrator2/1 -> Degrees to Radians1/1
  vel angular/1 -> Transfer Fcn1/1
  Degrees to Radians1/1 -> posicion angular/1

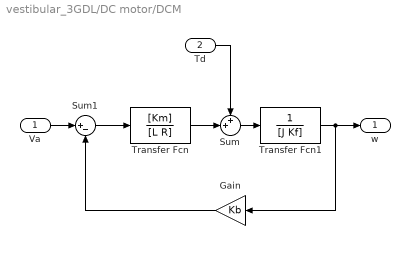
== system vestibular_3GDL/DC motor/DCM ==
  Va : Inport
  Td : Inport  Port=2
  Gain : Gain  Gain=Kb
  Sum : Sum  Inputs=++|
  Sum1 : Sum  Inputs=|+-
  Transfer Fcn : TransferFcn  Numerator=[Km]  Denominator=[L R]
  Transfer Fcn1 : TransferFcn  Denominator=[J Kf]
  w : Outport
  wires:
  Transfer Fcn/1 -> Sum/2
  Gain/1 -> Sum1/2
  Sum1/1 -> Transfer Fcn/1
  Sum/1 -> Transfer Fcn1/1
  Transfer Fcn1/1 -> Gain/1, w/1
  Td/1 -> Sum/1
  Va/1 -> Sum1/1

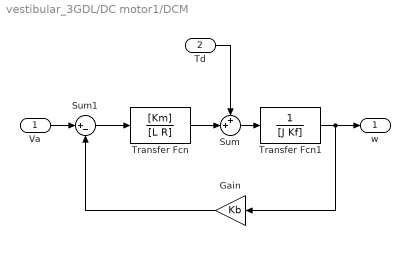
== system vestibular_3GDL/DC motor1/DCM ==
  Va : Inport
  Td : Inport  Port=2
  Gain : Gain  Gain=Kb
  Sum : Sum  Inputs=++|
  Sum1 : Sum  Inputs=|+-
  Transfer Fcn : TransferFcn  Numerator=[Km]  Denominator=[L R]
  Transfer Fcn1 : TransferFcn  Denominator=[J Kf]
  w : Outport
  wires:
  Va/1 -> Sum1/1
  Td/1 -> Sum/1
  Transfer Fcn1/1 -> w/1, Gain/1
  Sum/1 -> Transfer Fcn1/1
  Sum1/1 -> Transfer Fcn/1
  Gain/1 -> Sum1/2
  Transfer Fcn/1 -> Sum/2

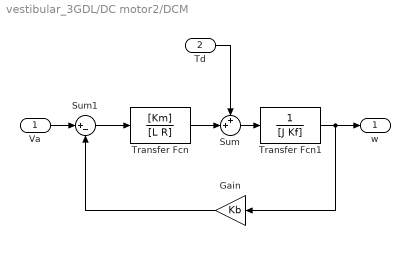
== system vestibular_3GDL/DC motor2/DCM ==
  Va : Inport
  Td : Inport  Port=2
  Gain : Gain  Gain=Kb
  Sum : Sum  Inputs=++|
  Sum1 : Sum  Inputs=|+-
  Transfer Fcn : TransferFcn  Numerator=[Km]  Denominator=[L R]
  Transfer Fcn1 : TransferFcn  Denominator=[J Kf]
  w : Outport
  wires:
  Va/1 -> Sum1/1
  Td/1 -> Sum/1
  Transfer Fcn1/1 -> w/1, Gain/1
  Sum/1 -> Transfer Fcn1/1
  Sum1/1 -> Transfer Fcn/1
  Gain/1 -> Sum1/2
  Transfer Fcn/1 -> Sum/2

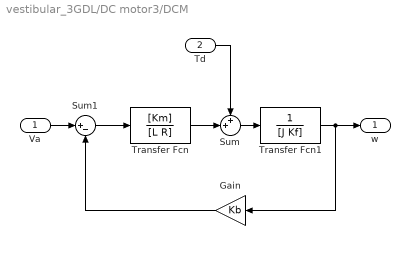
== system vestibular_3GDL/DC motor3/DCM ==
  Va : Inport
  Td : Inport  Port=2
  Gain : Gain  Gain=Kb
  Sum : Sum  Inputs=++|
  Sum1 : Sum  Inputs=|+-
  Transfer Fcn : TransferFcn  Numerator=[Km]  Denominator=[L R]
  Transfer Fcn1 : TransferFcn  Denominator=[J Kf]
  w : Outport
  wires:
  Transfer Fcn/1 -> Sum/2
  Gain/1 -> Sum1/2
  Sum1/1 -> Transfer Fcn/1
  Sum/1 -> Transfer Fcn1/1
  Transfer Fcn1/1 -> Gain/1, w/1
  Td/1 -> Sum/1
  Va/1 -> Sum1/1
